simulink model "step"  (R2024a)
settings: Solver=VariableStepAuto  StartTime=0.0  StopTime=10.0  RelTol=1e-3
settings Model: Creator=tusha  LastModifiedBy=tusha

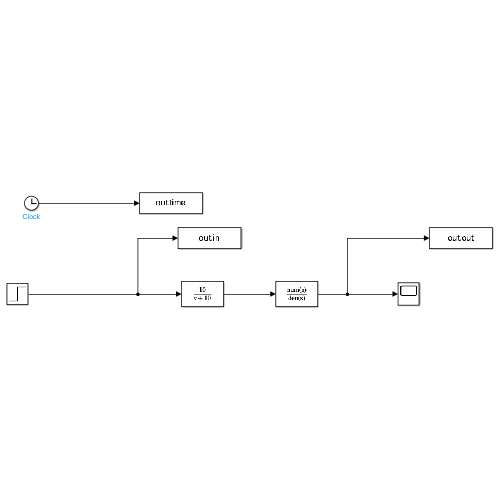
[thumbnail: Simulink's stored preview of the top-level diagram]
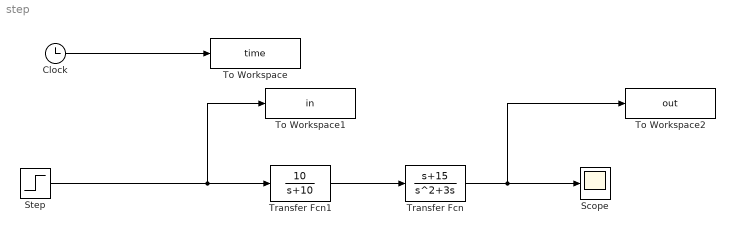
== system step ==
  Clock : Clock
  Scope : Scope
  Step : Step  SampleTime=0
  To Workspace : ToWorkspace  VariableName=time  SaveFormat=Timeseries
  To Workspace1 : ToWorkspace  VariableName=in  SaveFormat=Timeseries  SampleTime=-1
  To Workspace2 : ToWorkspace  VariableName=out  SaveFormat=Timeseries  SampleTime=-1
  Transfer Fcn : TransferFcn  Numerator=[1 15]  Denominator=[1 3 0]
  Transfer Fcn1 : TransferFcn  Numerator=[10]  Denominator=[1 10]
  wires:
  Clock/1 -> To Workspace/1
  Transfer Fcn/1 -> To Workspace2/1, Scope/1
  Step/1 -> To Workspace1/1, Transfer Fcn1/1
  Transfer Fcn1/1 -> Transfer Fcn/1
